simulink model "SWC_Diag_AFE"  (R2022b)
settings: configuration reference "DC_DC_Charger_Configuration" (kept outside this file)
libraries: common_lib x8
settings Model: DataDictionary=SWC_Diag_AFE.sldd  ExtModeTrigDuration=8  Creator=E0654638  LastModifiedBy=E0660158
settings ConfigSetRef: SourceName=DC_DC_Charger_Configuration

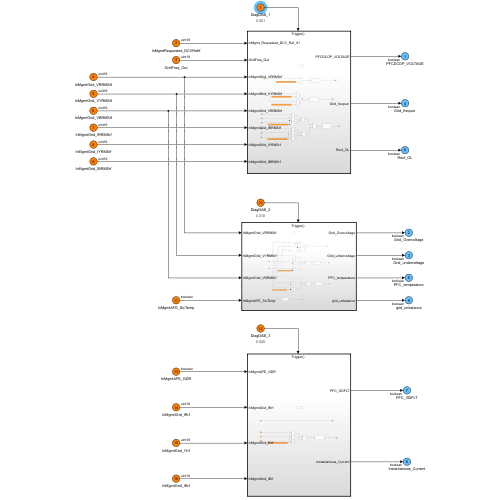
[thumbnail: Simulink's stored preview of the top-level diagram]
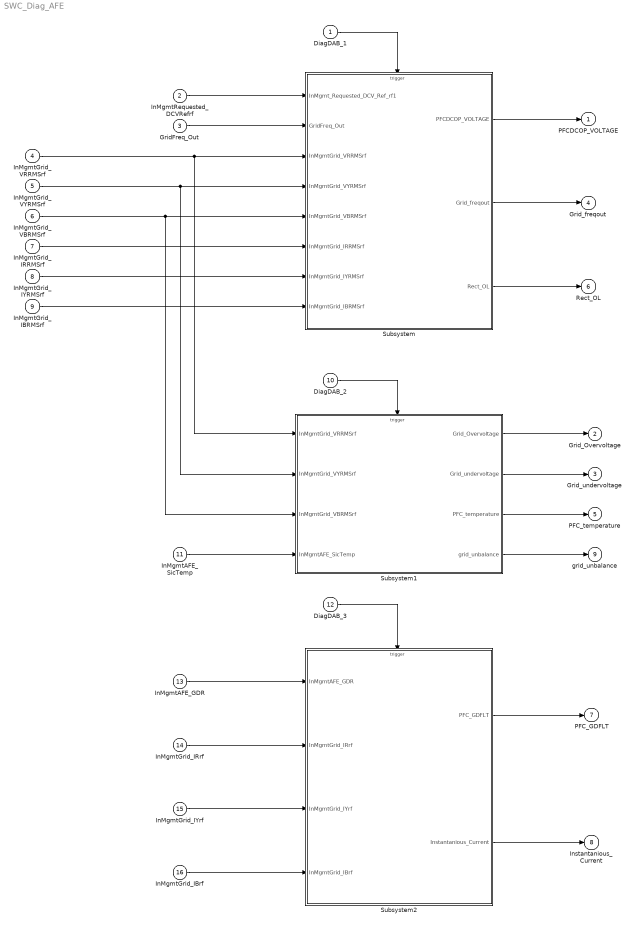
== system SWC_Diag_AFE ==
  DiagDAB_1 : Inport  Description=Inverter HVDC voltage  OutMin=0  OutMax=1000  PortDimensions=1  SampleTime=0.001  OutputFunctionCall=on
      settings: AttributesFormatString=%<SampleTime>
  InMgmtRequested_DCVRefrf : Inport  Port=2  OutDataTypeStr=uint16
  GridFreq_Out : Inport  Port=3  OutDataTypeStr=uint16
  InMgmtGrid_VRRMSrf : Inport  Port=4  OutDataTypeStr=uint16
  InMgmtGrid_VYRMSrf : Inport  Port=5  OutDataTypeStr=uint16
  InMgmtGrid_VBRMSrf : Inport  Port=6  OutDataTypeStr=uint16
  InMgmtGrid_IRRMSrf : Inport  Port=7  OutDataTypeStr=uint16
  InMgmtGrid_IYRMSrf : Inport  Port=8  OutDataTypeStr=uint16
  InMgmtGrid_IBRMSrf : Inport  Port=9  OutDataTypeStr=uint16
  DiagDAB_2 : Inport  Description=Inverter HVDC voltage  Port=10  OutMin=0  OutMax=1000  PortDimensions=1  SampleTime=0.010  OutputFunctionCall=on
      settings: AttributesFormatString=%<SampleTime>
  InMgmtAFE_SicTemp : Inport  Port=11  OutDataTypeStr=boolean
  DiagDAB_3 : Inport  Description=Inverter HVDC voltage  Port=12  OutMin=0  OutMax=1000  PortDimensions=1  SampleTime=0.025  OutputFunctionCall=on
      settings: AttributesFormatString=%<SampleTime>
  InMgmtAFE_GDR : Inport  Port=13  OutDataTypeStr=boolean
  InMgmtGrid_IRrf : Inport  Port=14  OutDataTypeStr=uint16
  InMgmtGrid_IYrf : Inport  Port=15  OutDataTypeStr=uint16
  InMgmtGrid_IBrf : Inport  Port=16  OutDataTypeStr=uint16
  Subsystem : Subsystem
  Subsystem1 : Subsystem
  Subsystem2 : Subsystem
  PFCDCOP_VOLTAGE : Outport  OutDataTypeStr=boolean  VectorParamsAs1DForOutWhenUnconnected=off
  Grid_Overvoltage : Outport  Port=2  OutDataTypeStr=boolean  VectorParamsAs1DForOutWhenUnconnected=off
  Grid_undervoltage : Outport  Port=3  OutDataTypeStr=boolean  VectorParamsAs1DForOutWhenUnconnected=off
  "Grid_freqout " : Outport  Port=4  OutDataTypeStr=boolean  VectorParamsAs1DForOutWhenUnconnected=off
  PFC_temperature : Outport  Port=5  OutDataTypeStr=boolean  VectorParamsAs1DForOutWhenUnconnected=off
  Rect_OL : Outport  Port=6  OutDataTypeStr=boolean  VectorParamsAs1DForOutWhenUnconnected=off
  PFC_GDFLT : Outport  Port=7  OutDataTypeStr=boolean  VectorParamsAs1DForOutWhenUnconnected=off
  Instantanious_Current : Outport  Port=8  OutDataTypeStr=boolean  VectorParamsAs1DForOutWhenUnconnected=off
  grid_unbalance : Outport  Port=9  OutDataTypeStr=boolean  VectorParamsAs1DForOutWhenUnconnected=off
  wires:
  InMgmtRequested_DCVRefrf/1 -> Subsystem/1(InMgmt_Requested_DCV_Ref_rf1)
  Subsystem/1(PFCDCOP_VOLTAGE) -> PFCDCOP_VOLTAGE/1
  DiagDAB_1/1 -> Subsystem/Trigger
  InMgmtGrid_VRRMSrf/1 -> Subsystem1/1(InMgmtGrid_VRRMSrf), Subsystem/3(InMgmtGrid_VRRMSrf)
  InMgmtGrid_VYRMSrf/1 -> Subsystem1/2(InMgmtGrid_VYRMSrf), Subsystem/4(InMgmtGrid_VYRMSrf)
  InMgmtGrid_VBRMSrf/1 -> Subsystem1/3(InMgmtGrid_VBRMSrf), Subsystem/5(InMgmtGrid_VBRMSrf)
  Subsystem1/1(Grid_Overvoltage) -> Grid_Overvoltage/1
  DiagDAB_2/1 -> Subsystem1/Trigger
  Subsystem1/2(Grid_undervoltage) -> Grid_undervoltage/1
  GridFreq_Out/1 -> Subsystem/2(GridFreq_Out)
  Subsystem/2("Grid_freqout ") -> "Grid_freqout "/1
  InMgmtAFE_SicTemp/1 -> Subsystem1/4(InMgmtAFE_SicTemp)
  Subsystem1/3(PFC_temperature) -> PFC_temperature/1
  Subsystem/3(Rect_OL) -> Rect_OL/1
  Subsystem2/2(Instantanious_Current) -> Instantanious_Current/1
  InMgmtGrid_IBRMSrf/1 -> Subsystem/8(InMgmtGrid_IBRMSrf)
  InMgmtGrid_IYRMSrf/1 -> Subsystem/7(InMgmtGrid_IYRMSrf)
  InMgmtGrid_IRRMSrf/1 -> Subsystem/6(InMgmtGrid_IRRMSrf)
  DiagDAB_3/1 -> Subsystem2/Trigger
  Subsystem2/1(PFC_GDFLT) -> PFC_GDFLT/1
  InMgmtAFE_GDR/1 -> Subsystem2/1(InMgmtAFE_GDR)
  Subsystem1/4(grid_unbalance) -> grid_unbalance/1
  InMgmtGrid_IRrf/1 -> Subsystem2/2(InMgmtGrid_IRrf)
  InMgmtGrid_IYrf/1 -> Subsystem2/3(InMgmtGrid_IYrf)
  InMgmtGrid_IBrf/1 -> Subsystem2/4(InMgmtGrid_IBrf)

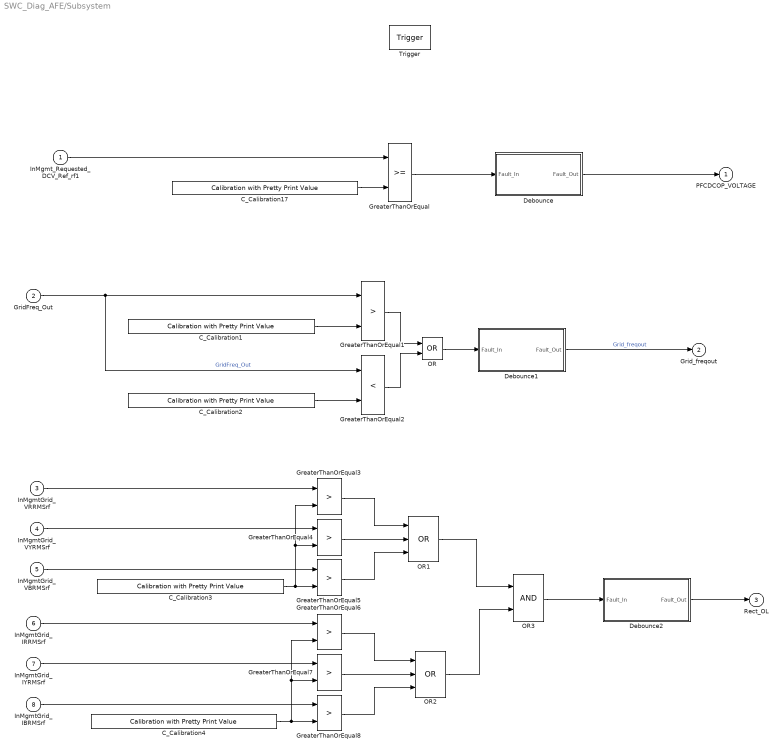
== system SWC_Diag_AFE/Subsystem ==
  InMgmt_Requested_DCV_Ref_rf1 : Inport
  GridFreq_Out : Inport  Port=2
  InMgmtGrid_VRRMSrf : Inport  Port=3
  InMgmtGrid_VYRMSrf : Inport  Port=4
  InMgmtGrid_VBRMSrf : Inport  Port=5
  InMgmtGrid_IRRMSrf : Inport  Port=6
  InMgmtGrid_IYRMSrf : Inport  Port=7
  InMgmtGrid_IBRMSrf : Inport  Port=8
  Trigger : TriggerPort  TriggerType=function-call  VariantControl=(inherit)  SampleTime=-1  PortDimensions=1
  C_Calibration1 : common_lib/IO/Calibration with Pretty Print Value  CalValue=GridFreq_UThd  scaling=None
      settings: SourceProductName=Common Library Blocks
  C_Calibration17 : common_lib/IO/Calibration with Pretty Print Value  CalValue=InMgmtRequestedDCVRef_UThd  scaling=None
      settings: SourceProductName=Common Library Blocks
  C_Calibration2 : common_lib/IO/Calibration with Pretty Print Value  CalValue=GridFreq_LThd  scaling=None
      settings: SourceProductName=Common Library Blocks
  C_Calibration3 : common_lib/IO/Calibration with Pretty Print Value  CalValue=InMgmt_GridVRMS_LTHD  scaling=None
      settings: SourceProductName=Common Library Blocks
  C_Calibration4 : common_lib/IO/Calibration with Pretty Print Value  CalValue=InMgmt_GridIRMS_UTHD  scaling=None
      settings: SourceProductName=Common Library Blocks
  Debounce : Subsystem
  Debounce1 : Subsystem
  Debounce2 : Subsystem
  GreaterThanOrEqual : RelationalOperator  OutDataTypeStr=boolean  RndMeth=Simplest  InputSameDT=off
  GreaterThanOrEqual{1,3..8} (7 alike) : RelationalOperator  Operator=>  OutDataTypeStr=boolean  RndMeth=Simplest  InputSameDT=off
  GreaterThanOrEqual2 : RelationalOperator  Operator=<  OutDataTypeStr=boolean  RndMeth=Simplest  InputSameDT=off
  OR : Logic  Operator=OR  AllPortsSameDT=off  OutDataTypeStr=boolean
  OR1 : Logic  Operator=OR  Inputs=3  AllPortsSameDT=off  OutDataTypeStr=boolean
  OR2 : Logic  Operator=OR  Inputs=3  AllPortsSameDT=off  OutDataTypeStr=boolean
  OR3 : Logic  AllPortsSameDT=off  OutDataTypeStr=boolean
  PFCDCOP_VOLTAGE : Outport  VectorParamsAs1DForOutWhenUnconnected=off
  "Grid_freqout " : Outport  Port=2  VectorParamsAs1DForOutWhenUnconnected=off
  Rect_OL : Outport  Port=3  VectorParamsAs1DForOutWhenUnconnected=off
  wires:
  Debounce/1(Fault_Out) -> PFCDCOP_VOLTAGE/1
  C_Calibration17/1 -> GreaterThanOrEqual/2
  GreaterThanOrEqual/1 -> Debounce/1(Fault_In)
  InMgmt_Requested_DCV_Ref_rf1/1 -> GreaterThanOrEqual/1
  GridFreq_Out/1 -> GreaterThanOrEqual2/1, GreaterThanOrEqual1/1  "GridFreq_Out"
  C_Calibration1/1 -> GreaterThanOrEqual1/2
  C_Calibration2/1 -> GreaterThanOrEqual2/2
  GreaterThanOrEqual1/1 -> OR/1
  GreaterThanOrEqual2/1 -> OR/2
  OR/1 -> Debounce1/1(Fault_In)
  Debounce1/1(Fault_Out) -> "Grid_freqout "/1  "Grid_freqout"
  InMgmtGrid_VRRMSrf/1 -> GreaterThanOrEqual3/1
  InMgmtGrid_VYRMSrf/1 -> GreaterThanOrEqual4/1
  InMgmtGrid_VBRMSrf/1 -> GreaterThanOrEqual5/1
  C_Calibration3/1 -> GreaterThanOrEqual5/2, GreaterThanOrEqual4/2, GreaterThanOrEqual3/2
  InMgmtGrid_IRRMSrf/1 -> GreaterThanOrEqual6/1
  InMgmtGrid_IYRMSrf/1 -> GreaterThanOrEqual7/1
  InMgmtGrid_IBRMSrf/1 -> GreaterThanOrEqual8/1
  C_Calibration4/1 -> GreaterThanOrEqual7/2, GreaterThanOrEqual6/2, GreaterThanOrEqual8/2
  GreaterThanOrEqual3/1 -> OR1/1
  GreaterThanOrEqual4/1 -> OR1/2
  GreaterThanOrEqual5/1 -> OR1/3
  GreaterThanOrEqual7/1 -> OR2/2
  GreaterThanOrEqual6/1 -> OR2/1
  GreaterThanOrEqual8/1 -> OR2/3
  OR1/1 -> OR3/1
  OR2/1 -> OR3/2
  OR3/1 -> Debounce2/1(Fault_In)
  Debounce2/1(Fault_Out) -> Rect_OL/1

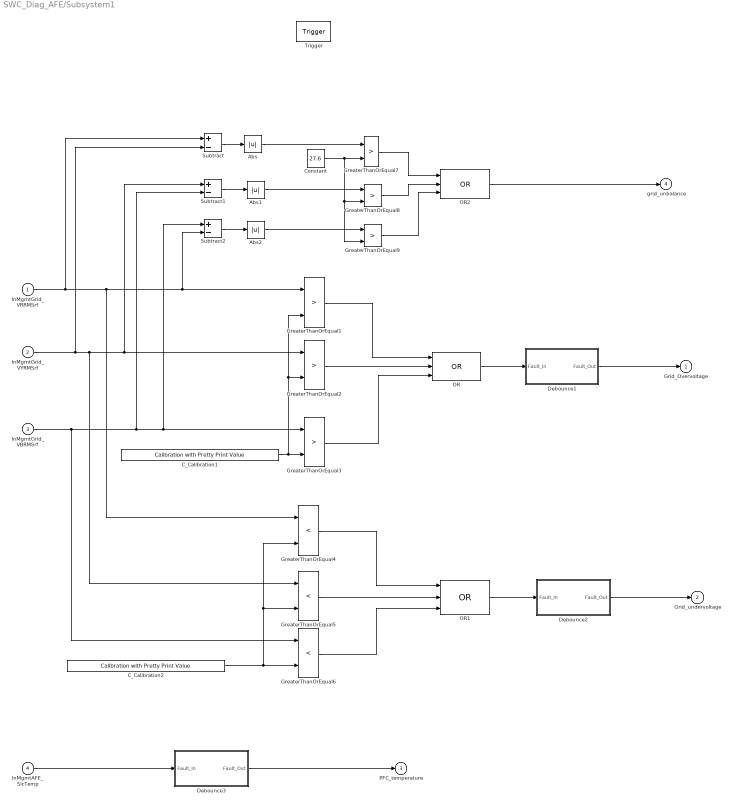
== system SWC_Diag_AFE/Subsystem1 ==
  InMgmtGrid_VRRMSrf : Inport
  InMgmtGrid_VYRMSrf : Inport  Port=2
  InMgmtGrid_VBRMSrf : Inport  Port=3
  InMgmtAFE_SicTemp : Inport  Port=4
  Trigger : TriggerPort  TriggerType=function-call  VariantControl=(inherit)  SampleTime=-1  PortDimensions=1
  Abs : Abs  SaturateOnIntegerOverflow=off
  Abs1 : Abs  SaturateOnIntegerOverflow=off
  Abs2 : Abs  SaturateOnIntegerOverflow=off
  C_Calibration1 : common_lib/IO/Calibration with Pretty Print Value  CalValue=InMgmtGridVRYBRMS_UThd  scaling=None
      settings: SourceProductName=Common Library Blocks
  C_Calibration2 : common_lib/IO/Calibration with Pretty Print Value  CalValue=InMgmtGridVRYBRMS_LThd  scaling=None
      settings: SourceProductName=Common Library Blocks
  Constant : Constant  Value=27.6
  Debounce1 : Subsystem
  Debounce2 : Subsystem
  Debounce3 : Subsystem
  GreaterThanOrEqual{1..3,7..9} (6 alike) : RelationalOperator  Operator=>  OutDataTypeStr=boolean  RndMeth=Simplest  InputSameDT=off
  GreaterThanOrEqual4 : RelationalOperator  Operator=<  OutDataTypeStr=boolean  RndMeth=Simplest  InputSameDT=off
  GreaterThanOrEqual5 : RelationalOperator  Operator=<  OutDataTypeStr=boolean  RndMeth=Simplest  InputSameDT=off
  GreaterThanOrEqual6 : RelationalOperator  Operator=<  OutDataTypeStr=boolean  RndMeth=Simplest  InputSameDT=off
  OR : Logic  Operator=OR  Inputs=3  AllPortsSameDT=off  OutDataTypeStr=boolean
  OR1 : Logic  Operator=OR  Inputs=3  AllPortsSameDT=off  OutDataTypeStr=boolean
  OR2 : Logic  Operator=OR  Inputs=3  AllPortsSameDT=off  OutDataTypeStr=boolean
  Subtract : Sum  Inputs=+-
  Subtract1 : Sum  Inputs=+-
  Subtract2 : Sum  Inputs=+-
  Grid_Overvoltage : Outport  VectorParamsAs1DForOutWhenUnconnected=off
  Grid_undervoltage : Outport  Port=2  VectorParamsAs1DForOutWhenUnconnected=off
  PFC_temperature : Outport  Port=3  VectorParamsAs1DForOutWhenUnconnected=off
  grid_unbalance : Outport  Port=4  VectorParamsAs1DForOutWhenUnconnected=off
  wires:
  C_Calibration1/1 -> GreaterThanOrEqual1/2, GreaterThanOrEqual2/2, GreaterThanOrEqual3/2
  GreaterThanOrEqual2/1 -> OR/2
  GreaterThanOrEqual3/1 -> OR/3
  GreaterThanOrEqual1/1 -> OR/1
  InMgmtGrid_VRRMSrf/1 -> Subtract/1, GreaterThanOrEqual4/1, Subtract2/2, GreaterThanOrEqual1/1
  OR/1 -> Debounce1/1(Fault_In)
  InMgmtGrid_VYRMSrf/1 -> Subtract/2, GreaterThanOrEqual5/1, Subtract1/1, GreaterThanOrEqual2/1
  Debounce1/1(Fault_Out) -> Grid_Overvoltage/1
  InMgmtGrid_VBRMSrf/1 -> GreaterThanOrEqual6/1, Subtract1/2, Subtract2/1, GreaterThanOrEqual3/1
  C_Calibration2/1 -> GreaterThanOrEqual4/2, GreaterThanOrEqual5/2, GreaterThanOrEqual6/2
  GreaterThanOrEqual4/1 -> OR1/1
  GreaterThanOrEqual5/1 -> OR1/2
  GreaterThanOrEqual6/1 -> OR1/3
  OR1/1 -> Debounce2/1(Fault_In)
  Debounce2/1(Fault_Out) -> Grid_undervoltage/1
  InMgmtAFE_SicTemp/1 -> Debounce3/1(Fault_In)
  Debounce3/1(Fault_Out) -> PFC_temperature/1
  Subtract/1 -> Abs/1
  Constant/1 -> GreaterThanOrEqual9/2, GreaterThanOrEqual8/2, GreaterThanOrEqual7/2
  Abs/1 -> GreaterThanOrEqual7/1
  GreaterThanOrEqual7/1 -> OR2/1
  OR2/1 -> grid_unbalance/1
  Subtract1/1 -> Abs1/1
  Subtract2/1 -> Abs2/1
  Abs1/1 -> GreaterThanOrEqual8/1
  Abs2/1 -> GreaterThanOrEqual9/1
  GreaterThanOrEqual8/1 -> OR2/2
  GreaterThanOrEqual9/1 -> OR2/3

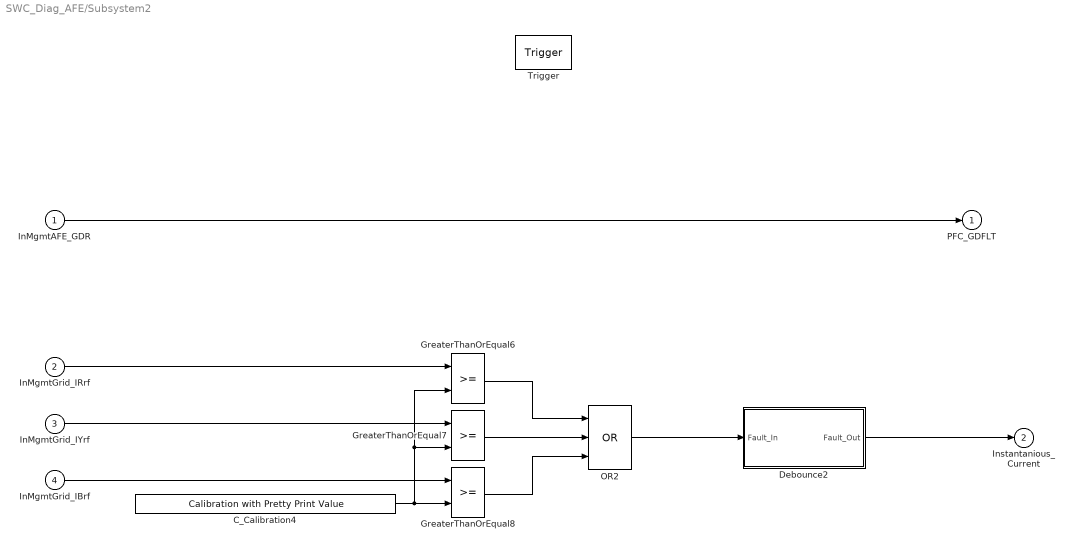
== system SWC_Diag_AFE/Subsystem2 ==
  InMgmtAFE_GDR : Inport
  InMgmtGrid_IRrf : Inport  Port=2
  InMgmtGrid_IYrf : Inport  Port=3
  InMgmtGrid_IBrf : Inport  Port=4
  Trigger : TriggerPort  TriggerType=function-call  VariantControl=(inherit)  SampleTime=-1  PortDimensions=1
  C_Calibration4 : common_lib/IO/Calibration with Pretty Print Value  CalValue=InMgmtGridI_UTHD  scaling=None
      settings: SourceProductName=Common Library Blocks
  Debounce2 : Subsystem
  GreaterThanOrEqual6 : RelationalOperator  OutDataTypeStr=boolean  RndMeth=Simplest  InputSameDT=off
  GreaterThanOrEqual7 : RelationalOperator  OutDataTypeStr=boolean  RndMeth=Simplest  InputSameDT=off
  GreaterThanOrEqual8 : RelationalOperator  OutDataTypeStr=boolean  RndMeth=Simplest  InputSameDT=off
  OR2 : Logic  Operator=OR  Inputs=3  AllPortsSameDT=off  OutDataTypeStr=boolean
  PFC_GDFLT : Outport  VectorParamsAs1DForOutWhenUnconnected=off
  Instantanious_Current : Outport  Port=2  VectorParamsAs1DForOutWhenUnconnected=off
  wires:
  Debounce2/1(Fault_Out) -> Instantanious_Current/1
  OR2/1 -> Debounce2/1(Fault_In)
  GreaterThanOrEqual8/1 -> OR2/3
  GreaterThanOrEqual6/1 -> OR2/1
  GreaterThanOrEqual7/1 -> OR2/2
  C_Calibration4/1 -> GreaterThanOrEqual8/2, GreaterThanOrEqual6/2, GreaterThanOrEqual7/2
  InMgmtGrid_IBrf/1 -> GreaterThanOrEqual8/1
  InMgmtGrid_IYrf/1 -> GreaterThanOrEqual7/1
  InMgmtGrid_IRrf/1 -> GreaterThanOrEqual6/1
  InMgmtAFE_GDR/1 -> PFC_GDFLT/1

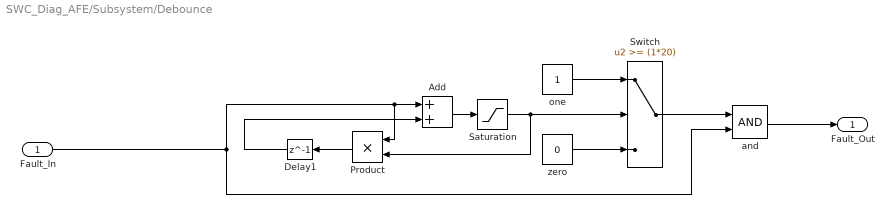
== system SWC_Diag_AFE/Subsystem/Debounce ==
  Fault_In : Inport
  Add : Sum
  Delay1 : Delay  DelayLength=1
  Product : Product
  Saturation : Saturate  UpperLimit=(1*20)+1  LowerLimit=0
  Switch : Switch  Threshold=(1*20)  SaturateOnIntegerOverflow=off  InputSameDT=off
  and : Logic  AllPortsSameDT=off  OutDataTypeStr=boolean
  one : Constant
  zero : Constant  Value=0
  Fault_Out : Outport  VectorParamsAs1DForOutWhenUnconnected=off
  wires:
  Fault_In/1 -> Add/1, Product/1, and/2
  Product/1 -> Delay1/1
  Saturation/1 -> Switch/2, Product/2
  Add/1 -> Saturation/1
  zero/1 -> Switch/3
  one/1 -> Switch/1
  Delay1/1 -> Add/2
  Switch/1 -> and/1
  and/1 -> Fault_Out/1

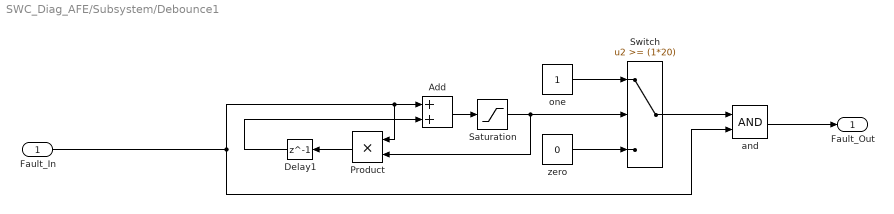
== system SWC_Diag_AFE/Subsystem/Debounce1 ==
  Fault_In : Inport
  Add : Sum
  Delay1 : Delay  DelayLength=1
  Product : Product
  Saturation : Saturate  UpperLimit=(1*20)+1  LowerLimit=0
  Switch : Switch  Threshold=(1*20)  SaturateOnIntegerOverflow=off  InputSameDT=off
  and : Logic  AllPortsSameDT=off  OutDataTypeStr=boolean
  one : Constant
  zero : Constant  Value=0
  Fault_Out : Outport  VectorParamsAs1DForOutWhenUnconnected=off
  wires:
  and/1 -> Fault_Out/1
  Switch/1 -> and/1
  Delay1/1 -> Add/2
  one/1 -> Switch/1
  zero/1 -> Switch/3
  Add/1 -> Saturation/1
  Saturation/1 -> Product/2, Switch/2
  Product/1 -> Delay1/1
  Fault_In/1 -> and/2, Product/1, Add/1

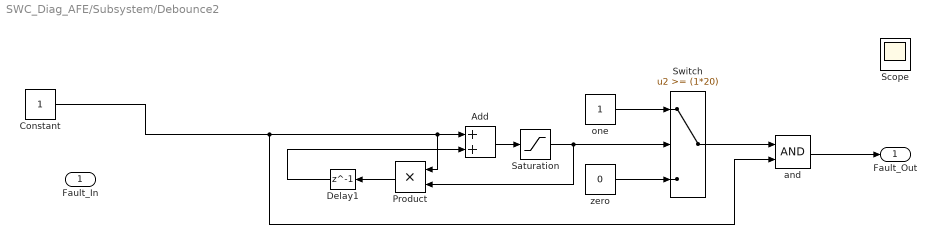
== system SWC_Diag_AFE/Subsystem/Debounce2 ==
  Fault_In : Inport
  Add : Sum
  Constant : Constant
  Delay1 : Delay  DelayLength=1
  Product : Product
  Saturation : Saturate  UpperLimit=(1*20)+1  LowerLimit=0
  Scope : Scope
  Switch : Switch  Threshold=(1*20)  SaturateOnIntegerOverflow=off  InputSameDT=off
  and : Logic  AllPortsSameDT=off  OutDataTypeStr=boolean
  one : Constant
  zero : Constant  Value=0
  Fault_Out : Outport  VectorParamsAs1DForOutWhenUnconnected=off
  wires:
  Constant/1 -> and/2, Add/1, Product/1
  Product/1 -> Delay1/1
  Saturation/1 -> Switch/2, Product/2
  Add/1 -> Saturation/1
  zero/1 -> Switch/3
  one/1 -> Switch/1
  Delay1/1 -> Add/2
  Switch/1 -> and/1
  and/1 -> Fault_Out/1

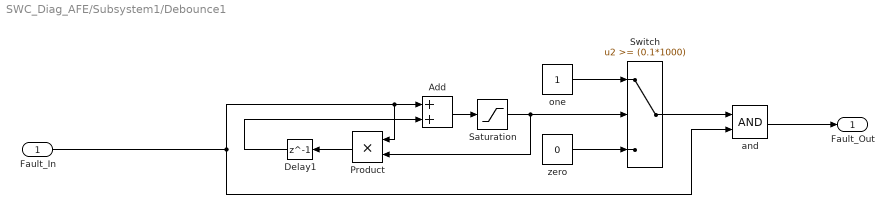
== system SWC_Diag_AFE/Subsystem1/Debounce1 ==
  Fault_In : Inport
  Add : Sum
  Delay1 : Delay  DelayLength=1
  Product : Product
  Saturation : Saturate  UpperLimit=(0.1*1000)+1  LowerLimit=0
  Switch : Switch  Threshold=(0.1*1000)  SaturateOnIntegerOverflow=off  InputSameDT=off
  and : Logic  AllPortsSameDT=off  OutDataTypeStr=boolean
  one : Constant
  zero : Constant  Value=0
  Fault_Out : Outport  VectorParamsAs1DForOutWhenUnconnected=off
  wires:
  and/1 -> Fault_Out/1
  Switch/1 -> and/1
  Delay1/1 -> Add/2
  one/1 -> Switch/1
  zero/1 -> Switch/3
  Add/1 -> Saturation/1
  Saturation/1 -> Product/2, Switch/2
  Product/1 -> Delay1/1
  Fault_In/1 -> and/2, Product/1, Add/1

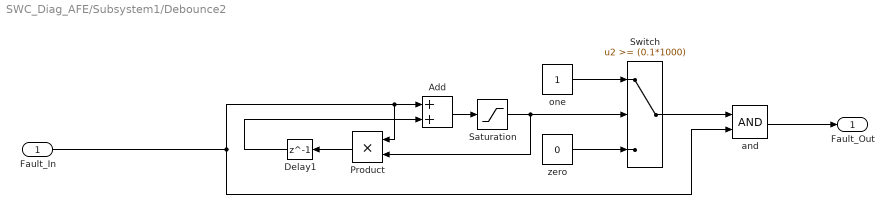
== system SWC_Diag_AFE/Subsystem1/Debounce2 ==
  Fault_In : Inport
  Add : Sum
  Delay1 : Delay  DelayLength=1
  Product : Product
  Saturation : Saturate  UpperLimit=(0.1*1000)+1  LowerLimit=0
  Switch : Switch  Threshold=(0.1*1000)  SaturateOnIntegerOverflow=off  InputSameDT=off
  and : Logic  AllPortsSameDT=off  OutDataTypeStr=boolean
  one : Constant
  zero : Constant  Value=0
  Fault_Out : Outport  VectorParamsAs1DForOutWhenUnconnected=off
  wires:
  Fault_In/1 -> Add/1, Product/1, and/2
  Product/1 -> Delay1/1
  Saturation/1 -> Switch/2, Product/2
  Add/1 -> Saturation/1
  zero/1 -> Switch/3
  one/1 -> Switch/1
  Delay1/1 -> Add/2
  Switch/1 -> and/1
  and/1 -> Fault_Out/1

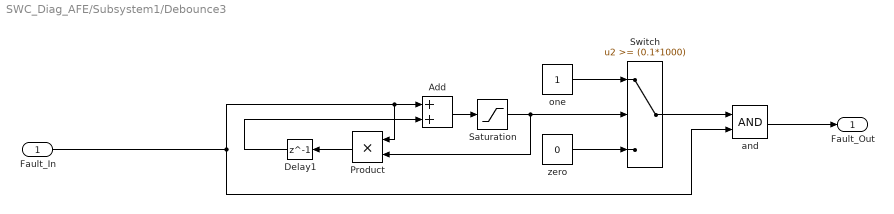
== system SWC_Diag_AFE/Subsystem1/Debounce3 ==
  Fault_In : Inport
  Add : Sum
  Delay1 : Delay  DelayLength=1
  Product : Product
  Saturation : Saturate  UpperLimit=(0.1*1000)+1  LowerLimit=0
  Switch : Switch  Threshold=(0.1*1000)  SaturateOnIntegerOverflow=off  InputSameDT=off
  and : Logic  AllPortsSameDT=off  OutDataTypeStr=boolean
  one : Constant
  zero : Constant  Value=0
  Fault_Out : Outport  VectorParamsAs1DForOutWhenUnconnected=off
  wires:
  and/1 -> Fault_Out/1
  Switch/1 -> and/1
  Delay1/1 -> Add/2
  one/1 -> Switch/1
  zero/1 -> Switch/3
  Add/1 -> Saturation/1
  Saturation/1 -> Product/2, Switch/2
  Product/1 -> Delay1/1
  Fault_In/1 -> and/2, Product/1, Add/1

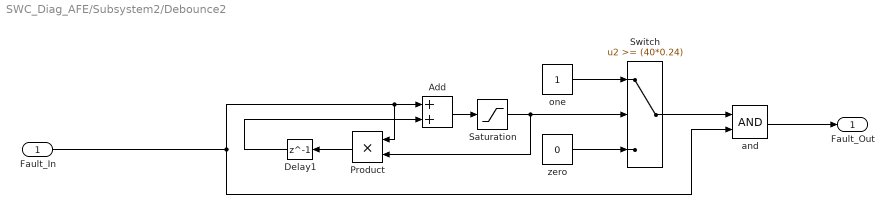
== system SWC_Diag_AFE/Subsystem2/Debounce2 ==
  Fault_In : Inport
  Add : Sum
  Delay1 : Delay  DelayLength=1
  Product : Product
  Saturation : Saturate  UpperLimit=(40*0.24)+1  LowerLimit=0
  Switch : Switch  Threshold=(40*0.24)  SaturateOnIntegerOverflow=off  InputSameDT=off
  and : Logic  AllPortsSameDT=off  OutDataTypeStr=boolean
  one : Constant
  zero : Constant  Value=0
  Fault_Out : Outport  VectorParamsAs1DForOutWhenUnconnected=off
  wires:
  and/1 -> Fault_Out/1
  Switch/1 -> and/1
  Delay1/1 -> Add/2
  one/1 -> Switch/1
  zero/1 -> Switch/3
  Add/1 -> Saturation/1
  Saturation/1 -> Product/2, Switch/2
  Product/1 -> Delay1/1
  Fault_In/1 -> and/2, Product/1, Add/1
